simulink model "cascaded_with_coading_singlephase_PD"  (R2022b)
settings: Solver=ode3  StartTime=0.0  StopTime=0.5  FixedStep=5e-5  RelTol=1e-3
libraries: spsIGBTDiodeLib x8, simulink x4, spsDCVoltageSourceLib x2, spsVoltageMeasurementLib x1, sps_lib x1
settings Model: Creator=gudel  LastModifiedBy=gudel

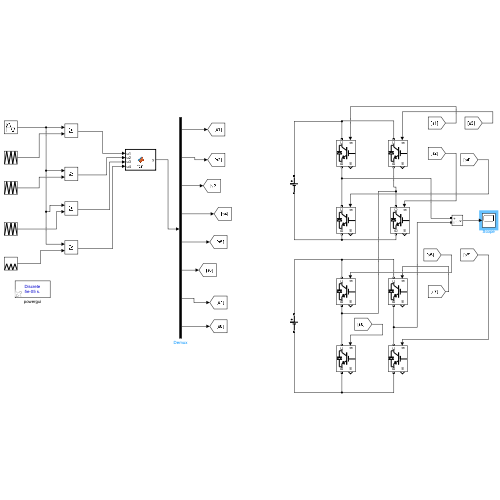
[thumbnail: Simulink's stored preview of the top-level diagram]
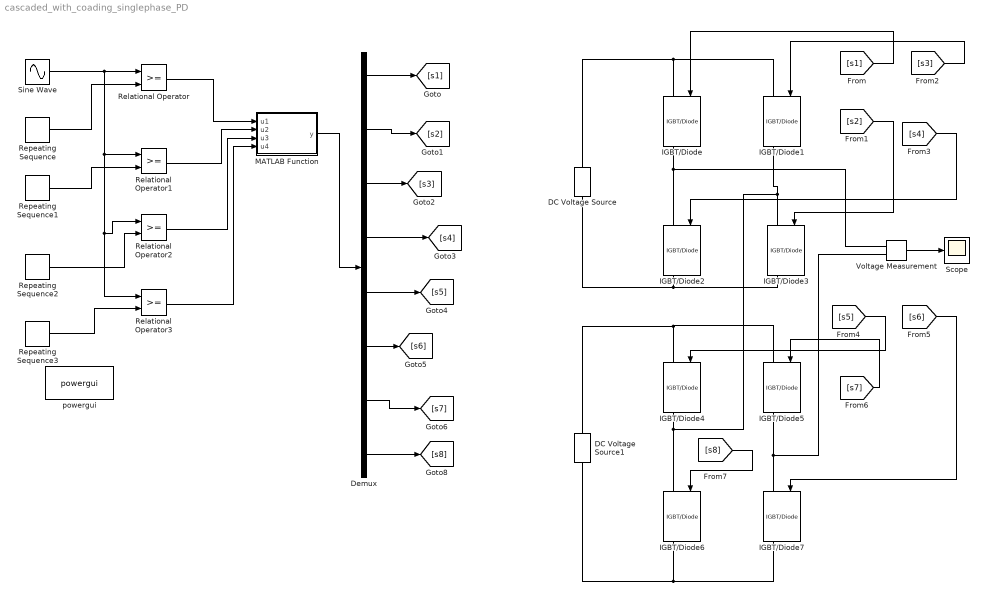
== system cascaded_with_coading_singlephase_PD ==
  DC Voltage Source : spsDCVoltageSourceLib/DC Voltage Source  Amplitude=100  Measurements=Voltage
  DC Voltage Source1 : spsDCVoltageSourceLib/DC Voltage Source  Amplitude=100  Measurements=Voltage
  Demux : Demux  Outputs=8
  IGBT/Diode{,1..7} (8 alike) : spsIGBTDiodeLib/IGBT//Diode  Ron=1e-3  Rs=1e5  Cs=inf  Measurements=on
  MATLAB Function : MATLAB Function  TreatAsAtomicUnit=on
  Relational Operator{,1..3} (4 alike) : RelationalOperator  OutDataTypeStr=boolean  RndMeth=Simplest  InputSameDT=off
  Repeating Sequence : simulink/Sources/Repeating Sequence  rep_seq_t=[0 0.5 1]*1/2000  rep_seq_y=[0.5 1 0.5]
  Repeating Sequence1 : simulink/Sources/Repeating Sequence  rep_seq_t=[0 0.5 1]*1/2000  rep_seq_y=[0 0.5 0]
  Repeating Sequence2 : simulink/Sources/Repeating Sequence  rep_seq_t=[0 0.5 1]*1/2000  rep_seq_y=[-0.5 0 -0.5]
  Repeating Sequence3 : simulink/Sources/Repeating Sequence  rep_seq_t=[0 0.5 1]*1/2000  rep_seq_y=[-1 -0.5 -1]
  Scope : Scope
  Sine Wave : Sin  Frequency=2*pi*50  SampleTime=0
  Voltage Measurement : spsVoltageMeasurementLib/Voltage Measurement  PhasorSimulation=off  OutputType=Complex  PSBequivalent=0
  powergui : sps_lib/powergui  Priority=1  SimulationMode=Discrete  SampleTime=50e-6  frequency=60  Iterations=50  frequencyindice=0  Pbase=100e6  ErrMax=1e-4  UnitsV=kV  UnitsW=MW  buscounter=0  FunctionMessages=off  echomessages=off  EnableUseOfTLC=off  CurrentSourceSwitches=off  DisableSnubberDevices=off  DisableRonSwitches=off  DisableVfSwitches=off  DisplayEquations=off  AutomaticDiscreteSolvers=off  SolverType=Tustin/Backward Euler (TBE)  Interpol=off  ExternalGateDelay=off  methode=off  Ts=100  x0status=blocks  SPID=on  SwTol=0  HookPort=off  NonlinearTolerance=1e-4  nMaxIteration=100  ContinueOnMaxIteration=off  RestoreLinks=warning  ResistiveCurrentMeasurement=off  Frange=[0:2:500]  Ylog=off  Xlog=on  ShowGrid=off  save=off  variable=ZData  structure=0  ZoomFFT=off  StartTime=0.0  cycles=1  DisplayStyle=1  fundamental=60  FreqAxis=off  MaxFrequency=1000  frequencyindicesteady=1  RmsSteady=1  display=off
  wires:
  Sine Wave/1 -> Relational Operator3/1, Relational Operator2/1, Relational Operator1/1, Relational Operator/1
  Repeating Sequence/1 -> Relational Operator/2
  Repeating Sequence1/1 -> Relational Operator1/2
  Repeating Sequence2/1 -> Relational Operator2/2
  Repeating Sequence3/1 -> Relational Operator3/2
  Relational Operator/1 -> MATLAB Function/1(u1)
  Relational Operator1/1 -> MATLAB Function/2(u2)
  Relational Operator2/1 -> MATLAB Function/3(u3)
  Relational Operator3/1 -> MATLAB Function/4(u4)
  MATLAB Function/1(y) -> Demux/1
  Demux/1 -> [s1]
  Demux/2 -> [s2]
  Demux/3 -> [s3]
  Demux/4 -> [s4]
  Demux/5 -> [s5]
  Demux/6 -> [s6]
  Demux/7 -> [s7]
  Demux/8 -> [s8]
  [s1] -> IGBT/Diode/1
  [s2] -> IGBT/Diode3/1
  [s3] -> IGBT/Diode1/1
  [s4] -> IGBT/Diode2/1
  [s5] -> IGBT/Diode4/1
  [s6] -> IGBT/Diode7/1
  [s7] -> IGBT/Diode5/1
  [s8] -> IGBT/Diode6/1
  Voltage Measurement/1 -> Scope/1
  connections:
  IGBT/Diode/RConn1 -- Voltage Measurement/LConn1 -- IGBT/Diode2/LConn1
  IGBT/Diode4/RConn1 -- IGBT/Diode3/LConn1 -- IGBT/Diode1/RConn1 -- IGBT/Diode6/LConn1
  IGBT/Diode/LConn1 -- DC Voltage Source/RConn1 -- IGBT/Diode1/LConn1
  IGBT/Diode2/RConn1 -- DC Voltage Source/LConn1 -- IGBT/Diode3/RConn1
  IGBT/Diode4/LConn1 -- DC Voltage Source1/RConn1 -- IGBT/Diode5/LConn1
  IGBT/Diode6/RConn1 -- DC Voltage Source1/LConn1 -- IGBT/Diode7/RConn1
  IGBT/Diode5/RConn1 -- Voltage Measurement/LConn2 -- IGBT/Diode7/LConn1

== matlab function cascaded_with_coading_singlephase_PD/MATLAB Function ==
  data: u1 input; y output; u2 input; u3 input; u4 input
function y = fcn(u1,u2,u3,u4)
SUM_sum=u1+u2+u3+u4;
s1=0;
s2=0;
s3=0;
s4=0;
s5=0;
s6=0;
s7=0;
s8=0;
if (SUM_sum==4)
    s1=1;
s2=1;
s3=0;
s4=0;
s5=1;
s6=1;
s7=0;
s8=0;
elseif(SUM_sum==3)
    s1=1;
s2=1;
s3=0;
s4=0;
s5=1;
s6=0;
s7=1;
s8=0;
elseif(SUM_sum==2)
    s1=1;
s2=0;
s3=1;
s4=0;
s5=1;
s6=0;
s7=1;
s8=0;
elseif(SUM_sum==1)
    s1=0;
s2=0;
s3=1;
s4=1;
s5=1;
s6=0;
s7=1;
s8=0;
elseif(SUM_sum==0)
    s1=0;
s2=0;
s3=1;
s4=1;
s5=0;
s6=0;
s7=1;
s8=1;
end
y = [s1 s2 s3 s4 s5 s6 s7 s8];
